simulink model "ap_12BAdapted_with_contracts_AutoPilot_SLDV"  (R2019b)
settings: Solver=FixedStepDiscrete  StartTime=0.0  StopTime=500  FixedStep=Ts  RelTol=1e-3  EnableMultiTasking=on
model workspace (MAT data in the model file):
  ContractValidatorBlocksMap : containers.Map (value not decoded)
undefined symbols (not defined in the file): beaver_b, beaver_c, beaver_mass, beaver_S, Cl0, Cl_alpha2_dpt, Cl_beta, Cl_da, Cl_da_alpha, Cl_dr, Cl_p, Cl_r, Cm0, Cm_alpha, Cm_alpha2, Cm_beta2, Cm_de, Cm_df, Cm_dpt, Cm_q, Cm_r, Cn0, Cn_beta, Cn_beta3, Cn_da, Cn_dpt3, Cn_dr, Cn_p, Cn_q, Cn_r, ContractEnsureBlock, ContractRequireBlock, Cx0, Cx_alpha, Cx_alpha2, Cx_alpha3, Cx_df, Cx_df_alpha, Cx_dpt, Cx_dpt2_alpha, Cx_dr, Cx_q, Cy0, Cy_beta, Cy_da, Cy_dr, Cy_dr_alpha, Cy_p, Cy_r, Cz0, Cz_alpha, Cz_alpha3, Cz_de, Cz_de_beta, Cz_df, Cz_df_alpha, Cz_dpt, Cz_q, d2r, fin_act_1 ... (+25)
libraries: simulink x10, sldvlib x5, cocosimLibs x3
(part 2 of 4)

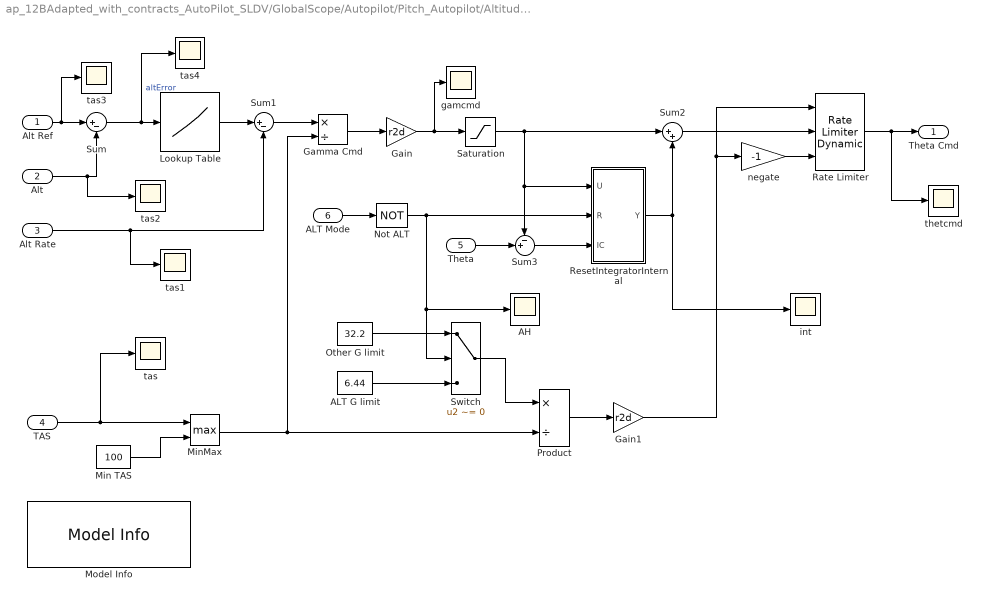
== system ap_12BAdapted_with_contracts_AutoPilot_SLDV/GlobalScope/Autopilot/Pitch_Autopilot/Altitude Mode ==
  Alt Ref : Inport  OutDataTypeStr=double  PortDimensions=1  SampleTime=1/40  Interpolate=off
  Alt : Inport  Port=2  OutDataTypeStr=double  PortDimensions=1  SampleTime=1/40  Interpolate=off
  Alt Rate : Inport  Port=3  OutDataTypeStr=double  PortDimensions=1  SampleTime=1/40  Interpolate=off
  TAS : Inport  Port=4  OutDataTypeStr=double  PortDimensions=1  SampleTime=1/40  Interpolate=off
  Theta : Inport  Port=5  OutDataTypeStr=double  PortDimensions=1  SampleTime=1/40  Interpolate=off
  ALT Mode : Inport  Port=6  OutDataTypeStr=boolean  PortDimensions=1  SampleTime=1/40  Interpolate=off
  AH : Scope
  ALT G limit : Constant  Value=6.44  OutDataTypeStr=double
  Gain : Gain  Gain=r2d
  Gain1 : Gain  Gain=r2d
  Gamma Cmd : Product  Inputs=*/  RndMeth=Zero
  Lookup Table : Lookup_n-D  NumberOfTableDimensions=1  BreakpointsForDimension1=[-544 -206 -116 -52 0 52 116 206]  Table=[-42 -26 -19 -13 0 13 19 26]  ExtrapMethod=Clip  RemoveProtectionInput=on  UseLastTableValue=on  RndMeth=Zero  FractionDataTypeStr=double  InputSameDT=on
  Min TAS : Constant  Value=100  OutDataTypeStr=double
  MinMax : MinMax  Function=max  Inputs=2  InputSameDT=on
  Model Info : simulink/Model-Wide Utilities/Model Info  Frame=on  DisplayStringWithTags=|  HorizontalTextAlignment=Left  LeftAlignmentValue=0.02
      | Altitude Mode
      | Author: %<LastModifiedBy>
      | Version: %<ModelVersion>
      | Date: %<LastModificationDate>
  Not ALT : Logic  Operator=NOT  IconShape=distinctive  AllPortsSameDT=off  OutDataTypeStr=boolean
  Other G limit : Constant  Value=32.2  OutDataTypeStr=double
  Product : Product  Inputs=*/  RndMeth=Zero
  Rate Limiter : simulink/Discontinuities/Rate Limiter Dynamic
      settings: SourceProductName=Simulink
  ResetIntegratorInternal : Subsystem
  Saturation : Saturate  UpperLimit=20  LowerLimit=-20
  Sum : Sum  Inputs=|+-
  Sum1 : Sum  Inputs=|+-
  Sum2 : Sum  Inputs=|++
  Sum3 : Sum  Inputs=-+|
  Switch : Switch  Criteria=u2 ~= 0
  gamcmd : Scope
  int : Scope
  negate : Gain  Gain=-1
  tas{,1..4} (5 alike) : Scope
  thetcmd : Scope
  Theta Cmd : Outport  OutDataTypeStr=double  PortDimensions=1  SampleTime=1/40  VectorParamsAs1DForOutWhenUnconnected=off
  wires:
  Other G limit/1 -> Switch/1
  Alt Ref/1 -> tas3/1, Sum/1
  Min TAS/1 -> MinMax/2
  Lookup Table/1 -> Sum1/1
  Rate Limiter/1 -> thetcmd/1, Theta Cmd/1
  negate/1 -> Rate Limiter/3
  MinMax/1 -> Gamma Cmd/2, Product/2
  Product/1 -> Gain1/1
  Gain1/1 -> negate/1, Rate Limiter/1
  Switch/1 -> Product/1
  ResetIntegratorInternal/1(Y) -> int/1, Sum2/2
  ALT G limit/1 -> Switch/3
  Sum2/1 -> Rate Limiter/2
  Theta/1 -> Sum3/2
  Sum/1 -> tas4/1, Lookup Table/1  "altError"
  Saturation/1 -> Sum3/1, ResetIntegratorInternal/1(U), Sum2/1
  ALT Mode/1 -> Not ALT/1
  Gain/1 -> gamcmd/1, Saturation/1
  Alt/1 -> tas2/1, Sum/2
  Sum1/1 -> Gamma Cmd/1
  Alt Rate/1 -> tas1/1, Sum1/2
  Gamma Cmd/1 -> Gain/1
  Not ALT/1 -> AH/1, Switch/2, ResetIntegratorInternal/2(R)
  Sum3/1 -> ResetIntegratorInternal/3(IC)
  TAS/1 -> tas/1, MinMax/1

== system ap_12BAdapted_with_contracts_AutoPilot_SLDV/GlobalScope/Autopilot/Pitch_Autopilot/Basic Pitch Mode ==
  note: Attitude Control using displacement, rate and integral
  Disp_Cmd : Inport  OutDataTypeStr=double  PortDimensions=1  SampleTime=1/40
  "Disp_FB " : Inport  Port=2  OutDataTypeStr=double  PortDimensions=1  SampleTime=1/40
  Rate_FB : Inport  Port=3  OutDataTypeStr=double  PortDimensions=1  SampleTime=1/40
  Engaged : Inport  Port=4  OutDataTypeStr=boolean  PortDimensions=1  SampleTime=1/40
  Cmd Limit : Saturate  UpperLimit=20  LowerLimit=-20
      settings: AttributesFormatString=%<LowerLimit> to %<UpperLimit> (deg)
  Disp Gain : Gain  Gain=2.0
  Disp Limit : Saturate  UpperLimit=20  LowerLimit=-20
      settings: AttributesFormatString=%<LowerLimit> to %<UpperLimit> (deg)
  Int Gain : Gain  Gain=0.5
  Model Info : simulink/Model-Wide Utilities/Model Info  Frame=on  DisplayStringWithTags=|  HorizontalTextAlignment=Left  LeftAlignmentValue=0.02
      | Attitude Controller
      | Author: %<LastModifiedBy>
      | Version: %<ModelVersion>
      | Date: %<LastModificationDate>
  Not engaged : Logic  Operator=NOT  IconShape=distinctive  AllPortsSameDT=off  OutDataTypeStr=boolean
  Rate Gain : Gain  Gain=2.0
  Rate Limit : Saturate  UpperLimit=3  LowerLimit=-3
      settings: AttributesFormatString=%<LowerLimit> to %<UpperLimit> (deg/sec)
  ResetIntegratorInternal : Subsystem
  Sum : Sum  Inputs=|+-
  Sum1 : Sum  Inputs=|+-
  Sum2 : Sum  Inputs=++|
  att : Scope
  q : Scope
  thet : Scope
  Surf_Cmd : Outport  OutDataTypeStr=double  PortDimensions=1  SampleTime=1/40  VectorParamsAs1DForOutWhenUnconnected=off
  wires:
  Rate Limit/1 -> Sum1/1
  ResetIntegratorInternal/1(Y) -> Sum2/1, att/1
  Sum2/1 -> Cmd Limit/1
  Disp Limit/1 -> Sum/1
  Engaged/1 -> Not engaged/1
  Cmd Limit/1 -> Surf_Cmd/1
  Disp_Cmd/1 -> Disp Limit/1
  Rate_FB/1 -> q/1, Sum1/2
  Sum1/1 -> Rate Gain/1, Int Gain/1
  Sum/1 -> Disp Gain/1
  Disp Gain/1 -> Rate Limit/1
  Rate Gain/1 -> Sum2/2
  "Disp_FB "/1 -> thet/1, Sum/2
  Not engaged/1 -> ResetIntegratorInternal/2(R)
  Int Gain/1 -> ResetIntegratorInternal/1(U)

== system ap_12BAdapted_with_contracts_AutoPilot_SLDV/GlobalScope/Autopilot/Pitch_Autopilot/Pitch Rate Feedback ==
  note: Pitch Rate Computation
  Phi : Inport
  Q : Inport  Port=2
  R : Inport  Port=3
  Gain : Gain  Gain=d2r
  Product : Product  RndMeth=Zero
  Product1 : Product  RndMeth=Zero
  Sum3 : Sum  Inputs=|++
  cos : Trigonometry  Operator=cos  OutputSignalType=real
  q : Scope
  sin : Trigonometry  OutputSignalType=real
  Pitch Rate : Outport  VectorParamsAs1DForOutWhenUnconnected=off
  wires:
  Phi/1 -> Gain/1
  Product/1 -> Sum3/2
  sin/1 -> Product/1
  R/1 -> Product/2
  Gain/1 -> sin/1, cos/1
  Product1/1 -> Sum3/1
  cos/1 -> Product1/1
  Q/1 -> Product1/2
  Sum3/1 -> q/1, Pitch Rate/1

== system ap_12BAdapted_with_contracts_AutoPilot_SLDV/GlobalScope/Autopilot/Pitch_Autopilot/Pitch Reference ==
  note: Pitch Reference
  Theta : Inport
  AP Eng : Inport  Port=2
  Pitch Wheel : Inport  Port=3
  Not engaged : Logic  Operator=NOT  IconShape=distinctive  AllPortsSameDT=off  OutDataTypeStr=boolean
  Sum3 : Sum  Inputs=|++
  latch : Subsystem
  Theta Ref : Outport  VectorParamsAs1DForOutWhenUnconnected=off
  wires:
  Not engaged/1 -> latch/2(E)
  latch/1(y) -> Sum3/1
  Theta/1 -> latch/1(u)
  AP Eng/1 -> Not engaged/1
  Sum3/1 -> Theta Ref/1
  Pitch Wheel/1 -> Sum3/2

== system ap_12BAdapted_with_contracts_AutoPilot_SLDV/GlobalScope/Autopilot/Roll_Autopilot/Basic Roll Mode ==
  note: Attitude Control using displacement, rate and integral
  Disp_Cmd : Inport  OutDataTypeStr=double  PortDimensions=1
  "Disp_FB " : Inport  Port=2  OutDataTypeStr=double  PortDimensions=1  SampleTime=1/40
  Rate_FB : Inport  Port=3  OutDataTypeStr=double  PortDimensions=1  SampleTime=1/40
  Engaged : Inport  Port=4  OutDataTypeStr=boolean  PortDimensions=1  SampleTime=1/40
  Cmd Limit : Saturate  UpperLimit=15  LowerLimit=-15
      settings: AttributesFormatString=%<LowerLimit> to %<UpperLimit> (deg)
  Disp Gain : Gain  Gain=1.0
  Disp Limit : Saturate  UpperLimit=30  LowerLimit=-30
      settings: AttributesFormatString=%<LowerLimit> to %<UpperLimit> (deg)
  Int Gain : Gain  Gain=1.0
  Model Info : simulink/Model-Wide Utilities/Model Info  Frame=on  DisplayStringWithTags=|  HorizontalTextAlignment=Left  LeftAlignmentValue=0.02
      | Attitude Controller
      | Author: %<LastModifiedBy>
      | Version: %<ModelVersion>
      | Date: %<LastModificationDate>
  Not engaged : Logic  Operator=NOT  IconShape=distinctive  AllPortsSameDT=off  OutDataTypeStr=boolean
  Rate Gain : Gain  Gain=3.0
  Rate Limit : Saturate  UpperLimit=6  LowerLimit=-6
      settings: AttributesFormatString=%<LowerLimit> to %<UpperLimit> (deg/sec)
  ResetIntegratorInternal : Subsystem
  Scope : Scope
  Scope1 : Scope
  Scope2 : Scope
  Sum : Sum  Inputs=|+-
  Sum1 : Sum  Inputs=|+-
  Sum2 : Sum  Inputs=++|
  Surf_Cmd : Outport  OutDataTypeStr=double  PortDimensions=1  SampleTime=1/40  VectorParamsAs1DForOutWhenUnconnected=off
  wires:
  Engaged/1 -> Not engaged/1
  Disp_Cmd/1 -> Disp Limit/1
  Rate Limit/1 -> Sum1/1
  ResetIntegratorInternal/1(Y) -> Sum2/1, Scope/1
  Not engaged/1 -> ResetIntegratorInternal/2(R)
  Rate_FB/1 -> Sum1/2
  Sum1/1 -> Int Gain/1, Scope1/1, Rate Gain/1
  Cmd Limit/1 -> Scope2/1, Surf_Cmd/1
  Rate Gain/1 -> Sum2/2
  Disp Gain/1 -> Rate Limit/1
  Sum/1 -> Disp Gain/1
  "Disp_FB "/1 -> Sum/2
  Disp Limit/1 -> Sum/1
  Sum2/1 -> Cmd Limit/1
  Int Gain/1 -> ResetIntegratorInternal/1(U)

== system ap_12BAdapted_with_contracts_AutoPilot_SLDV/GlobalScope/Autopilot/Roll_Autopilot/Heading Mode ==
  Psi Ref : Inport  OutDataTypeStr=double  PortDimensions=1  SampleTime=1/40  Interpolate=off
  Psi : Inport  Port=2  OutDataTypeStr=double  PortDimensions=1  SampleTime=1/40  Interpolate=off
  TAS : Inport  Port=3  OutDataTypeStr=double  PortDimensions=1  SampleTime=1/40  Interpolate=off
  Disp Gain : Gain  Gain=0.015
  Model Info : simulink/Model-Wide Utilities/Model Info  Frame=on  DisplayStringWithTags=|  HorizontalTextAlignment=Left  LeftAlignmentValue=0.02
      | Heading Mode
      | Author: %<LastModifiedBy>
      | Version: %<ModelVersion>
      | Date: %<LastModificationDate>
  Product : Product  RndMeth=Zero
  angle diff : Subsystem
  Phi Cmd : Outport  OutDataTypeStr=double  PortDimensions=1  SampleTime=1/40  VectorParamsAs1DForOutWhenUnconnected=off
  wires:
  Psi Ref/1 -> angle diff/1(plus)
  angle diff/1(diff) -> Disp Gain/1  "hdgError"
  TAS/1 -> Product/2
  Disp Gain/1 -> Product/1
  Psi/1 -> angle diff/2(minus)
  Product/1 -> Phi Cmd/1

== system ap_12BAdapted_with_contracts_AutoPilot_SLDV/GlobalScope/Autopilot/Roll_Autopilot/Roll Reference ==
  note: Roll Reference
  Phi : Inport
  AP eng : Inport  Port=2
  Turn Knob : Inport  Port=3
  Abs : Abs
  Not engaged : Logic  Operator=NOT  IconShape=distinctive  AllPortsSameDT=off  OutDataTypeStr=boolean
  Ref Threshold : RelationalOperator  OutDataTypeStr=boolean  RndMeth=Nearest  InputSameDT=on
  Ref Threshold1 : RelationalOperator  Operator=<=  OutDataTypeStr=boolean  RndMeth=Nearest  InputSameDT=on
  TK Threshold : RelationalOperator  Operator=<  OutDataTypeStr=boolean  RndMeth=Nearest  InputSameDT=on
  TK switch : Switch  Criteria=u2 ~= 0
  latch : Subsystem
  minus six : Constant  Value=-6
  or : Logic  Operator=OR  IconShape=distinctive  OutDataTypeStr=boolean
  ref switch : Switch  Criteria=u2 ~= 0
  six : Constant  Value=6
  three : Constant  Value=3  OutDataTypeStr=double
  zero : Constant  Value=0
  Phi Ref : Outport  VectorParamsAs1DForOutWhenUnconnected=off
  wires:
  minus six/1 -> Ref Threshold1/2
  Ref Threshold1/1 -> or/2
  Ref Threshold/1 -> or/1
  or/1 -> ref switch/2
  zero/1 -> ref switch/3
  six/1 -> Ref Threshold/2
  TK switch/1 -> Phi Ref/1
  AP eng/1 -> Not engaged/1
  Phi/1 -> Ref Threshold1/1, Ref Threshold/1, ref switch/1
  Abs/1 -> TK Threshold/1
  three/1 -> TK Threshold/2
  Turn Knob/1 -> Abs/1, TK switch/3
  TK Threshold/1 -> TK switch/2
  latch/1(y) -> TK switch/1
  ref switch/1 -> latch/1(u)
  Not engaged/1 -> latch/2(E)

== system ap_12BAdapted_with_contracts_AutoPilot_SLDV/GlobalScope/Autopilot/Yaw_damper/Basic Yaw Damper ==
  note: Basic Yaw Damper
  "Phi " : Inport
  R : Inport  Port=2
  TAS : Inport  Port=3
  Constant : Constant  Value=100
  MinMax : MinMax  Function=max  Inputs=2
  Model Info : simulink/Model-Wide Utilities/Model Info  Frame=on  DisplayStringWithTags=|  HorizontalTextAlignment=Left  LeftAlignmentValue=0.02
      | Yaw Damper
      | Author: %<LastModifiedBy>
      | Date: %<LastModificationDate>
      | Model Version: %<ModelVersion>
  Product : Product  Inputs=*/  RndMeth=Zero
  Rate Gain : Gain  Gain=1.0
  Rud Limit : Saturate  UpperLimit=25  LowerLimit=-25
      settings: AttributesFormatString=%<LowerLimit> to %<UpperLimit> (deg)
  Sum1 : Sum  Inputs=|+-
  gravity : Gain  Gain=32.2
  sin : Trigonometry
  Rud Cmd : Outport  VectorParamsAs1DForOutWhenUnconnected=off
  wires:
  R/1 -> Sum1/2
  Sum1/1 -> Rate Gain/1  "yawRate"
  Rud Limit/1 -> Rud Cmd/1
  Rate Gain/1 -> Rud Limit/1
  "Phi "/1 -> sin/1
  sin/1 -> gravity/1
  Product/1 -> Sum1/1
  gravity/1 -> Product/1
  MinMax/1 -> Product/2
  TAS/1 -> MinMax/1
  Constant/1 -> MinMax/2

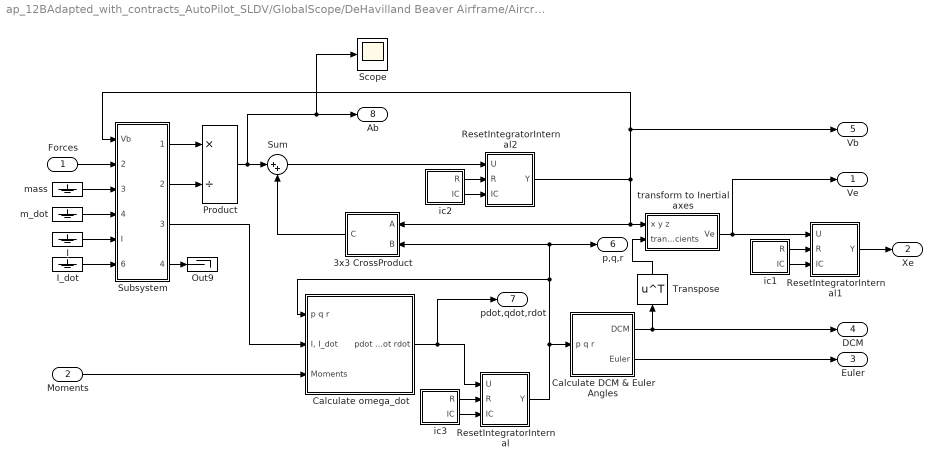
== system ap_12BAdapted_with_contracts_AutoPilot_SLDV/GlobalScope/DeHavilland Beaver Airframe/Aircraft Dynamics/6DoF (Quaternion) ==
  Forces : Inport
  Moments : Inport  Port=2
  3x3 CrossProduct : Subsystem
  Calculate DCM & Euler Angles : Subsystem
  Calculate omega_dot : Subsystem
  I : Ground
  I_dot : Ground
  Out9 : Terminator
  Product : Product  Inputs=*/  SaturateOnIntegerOverflow=on  OutDataTypeStr=Inherit: Same as first input
  ResetIntegratorInternal : Subsystem
  ResetIntegratorInternal1 : Subsystem
  ResetIntegratorInternal2 : Subsystem
  Scope : Scope
  Subsystem : Subsystem
  Sum : Sum  Inputs=|++  SaturateOnIntegerOverflow=on
  Transpose : Math  Operator=transpose  SaturateOnIntegerOverflow=on
  ic1 : Subsystem
  ic2 : Subsystem
  ic3 : Subsystem
  m_dot : Ground
  mass : Ground
  "transform to Inertial axes " : Subsystem
  Ve : Outport  VectorParamsAs1DForOutWhenUnconnected=off
  Xe : Outport  Port=2  VectorParamsAs1DForOutWhenUnconnected=off
  Euler : Outport  Port=3  VectorParamsAs1DForOutWhenUnconnected=off
  DCM : Outport  Port=4  VectorParamsAs1DForOutWhenUnconnected=off
  Vb : Outport  Port=5  VectorParamsAs1DForOutWhenUnconnected=off
  p,q,r : Outport  Port=6  VectorParamsAs1DForOutWhenUnconnected=off
  pdot,qdot,rdot : Outport  Port=7  VectorParamsAs1DForOutWhenUnconnected=off
  Ab : Outport  Port=8  VectorParamsAs1DForOutWhenUnconnected=off
  wires:
  Subsystem/1("forces ") -> Product/1
  I_dot/1 -> Subsystem/6(I_dot)
  I/1 -> Subsystem/5(I)
  Calculate omega_dot/1(pdot qdot rdot) -> pdot,qdot,rdot/1, ResetIntegratorInternal/1(U)
  Subsystem/4(Out9) -> Out9/1
  m_dot/1 -> Subsystem/4(m_dot)
  Subsystem/2(mass) -> Product/2
  mass/1 -> Subsystem/3("mass ")
  Transpose/1 -> "transform to Inertial axes "/2(transform coefficients)
  Calculate DCM & Euler Angles/1(DCM) -> DCM/1, Transpose/1
  Product/1 -> Scope/1, Ab/1, Sum/1
  Forces/1 -> Subsystem/2(forces)
  Moments/1 -> Calculate omega_dot/3(Moments)
  ResetIntegratorInternal1/1(Y) -> Xe/1
  Sum/1 -> ResetIntegratorInternal2/1(U)
  3x3 CrossProduct/1(C) -> Sum/2
  Calculate DCM & Euler Angles/2(Euler) -> Euler/1
  Subsystem/3("inertia, 0") -> Calculate omega_dot/2("I, I_dot")
  "transform to Inertial axes "/1(Ve) -> ResetIntegratorInternal1/1(U), Ve/1
  ResetIntegratorInternal/1(Y) -> Calculate DCM & Euler Angles/1(p q r), 3x3 CrossProduct/2(B), p,q,r/1, Calculate omega_dot/1(p q r)
  ic3/1(R) -> ResetIntegratorInternal/2(R)
  ic3/2(IC) -> ResetIntegratorInternal/3(IC)
  ic1/1(R) -> ResetIntegratorInternal1/2(R)
  ic1/2(IC) -> ResetIntegratorInternal1/3(IC)
  ic2/1(R) -> ResetIntegratorInternal2/2(R)
  ic2/2(IC) -> ResetIntegratorInternal2/3(IC)
  ResetIntegratorInternal2/1(Y) -> Subsystem/1(Vb), Vb/1, 3x3 CrossProduct/1(A), "transform to Inertial axes "/1(x y z)

== system ap_12BAdapted_with_contracts_AutoPilot_SLDV/GlobalScope/DeHavilland Beaver Airframe/Aircraft Dynamics/Total Forces and Moments ==
  EnvirBus : Inport
  Pilot : Inport  Port=2
  DCM : Inport  Port=3
  FltParams : Inport  Port=4
  Actuators : Subsystem
  Aerodynamics : Subsystem
  Bus Selector4 : BusSelector  OutputSignals=rho,g
  "Engine " : Subsystem
  Forces and Moments : Subsystem
  "Gravity " : Subsystem
  "Pilot " : InportShadow  Port=2
  Sum : Sum  Inputs=|++  SaturateOnIntegerOverflow=on  InputSameDT=on  OutDataTypeStr=Inherit: Same as first input
  Total Force : Outport  VectorParamsAs1DForOutWhenUnconnected=off
  Total Moment : Outport  Port=2  VectorParamsAs1DForOutWhenUnconnected=off
  wires:
  Forces and Moments/1(XYZ) -> Sum/1
  "Engine "/1(Engine Coefficients) -> Forces and Moments/3(Engine Coefficients)
  "Gravity "/1(Fgrav) -> Sum/2
  Aerodynamics/1(Aero Coefficients) -> Forces and Moments/1(Aero Coefficients)
  Pilot/1 -> Actuators/1(Pilot)
  Bus Selector4/1 -> "Engine "/3(rho)  "<rho>"
  DCM/1 -> "Gravity "/2(DCM)
  Bus Selector4/2 -> "Gravity "/1(g)  "<g>"
  Sum/1 -> Total Force/1  "Ftot"
  Forces and Moments/2(LMN) -> Total Moment/1  "Mtot"
  "Pilot "/1 -> "Engine "/2(Pilot)
  FltParams/1 -> Forces and Moments/2(Fltparams), "Engine "/1(Fltparams), Aerodynamics/2(FltParams)
  Actuators/1(uaero-out) -> Aerodynamics/1(Uaero)
  EnvirBus/1 -> Bus Selector4/1

== system ap_12BAdapted_with_contracts_AutoPilot_SLDV/GlobalScope/DeHavilland Beaver Airframe/Calculate Parameters/ Incidence, Sideslip, & Airspeed ==
  Vb : Inport
  Airspeed : Sqrt  AlgorithmType=Newton-Raphson  SaturateOnIntegerOverflow=on
  Incidence : Trigonometry  Operator=atan2
  Product : Product  Inputs=*/  SaturateOnIntegerOverflow=on  OutDataTypeStr=Inherit: Same as first input
  Sideslip : Trigonometry  Operator=asin
  Subsystem : Subsystem
  Subsystem1 : Subsystem
  dot : Subsystem
  Alpha : Outport  VectorParamsAs1DForOutWhenUnconnected=off
  Beta : Outport  Port=2  VectorParamsAs1DForOutWhenUnconnected=off
  V : Outport  Port=3  VectorParamsAs1DForOutWhenUnconnected=off
  wires:
  Sideslip/1 -> Beta/1
  Subsystem1/1(v) -> Product/1
  Product/1 -> Sideslip/1
  Subsystem/1(w) -> Incidence/1
  Subsystem/2(U) -> Incidence/2
  dot/1(dot) -> Airspeed/1
  Airspeed/1 -> V/1, Product/2
  Incidence/1 -> Alpha/1
  Vb/1 -> Subsystem/1(V), dot/1(Vb), Subsystem1/1(V)

== system ap_12BAdapted_with_contracts_AutoPilot_SLDV/GlobalScope/DeHavilland Beaver Airframe/Calculate Parameters/Dynamic Pressure ==
  Velocity : Inport
  Air Density : Inport  Port=2
  1/2rhoV^2 : Gain  Gain=0.5  SaturateOnIntegerOverflow=on  OutDataTypeStr=Inherit: Same as input  ParamDataTypeStr=Inherit: Same as input
  Product2 : Product  SaturateOnIntegerOverflow=on  InputSameDT=on  OutDataTypeStr=Inherit: Same as first input
  dot : Subsystem
  qbar : Outport  VectorParamsAs1DForOutWhenUnconnected=off
  wires:
  1/2rhoV^2/1 -> qbar/1
  Air Density/1 -> Product2/2
  dot/1(dot) -> Product2/1
  Product2/1 -> 1/2rhoV^2/1
  Velocity/1 -> dot/1(V)

== system ap_12BAdapted_with_contracts_AutoPilot_SLDV/GlobalScope/Sensors/Air Data Sensor/ Incidence, Sideslip, & Airspeed ==
  Vb : Inport
  Airspeed : Sqrt  AlgorithmType=Newton-Raphson  SaturateOnIntegerOverflow=on
  Gain : Gain  Gain=180/pi
  Gain1 : Gain  Gain=180/pi
  Incidence : Trigonometry  Operator=atan2
  Product : Product  Inputs=*/  SaturateOnIntegerOverflow=on  OutDataTypeStr=Inherit: Same as first input
  Scope : Scope
  Scope1 : Scope
  Sideslip : Trigonometry  Operator=asin
  Subsystem : Subsystem
  Subsystem1 : Subsystem
  dot : Subsystem
  Alpha : Outport  VectorParamsAs1DForOutWhenUnconnected=off
  Beta : Outport  Port=2  VectorParamsAs1DForOutWhenUnconnected=off
  V : Outport  Port=3  VectorParamsAs1DForOutWhenUnconnected=off
  wires:
  Sideslip/1 -> Gain1/1, Beta/1
  Subsystem1/1(v) -> Product/1
  Product/1 -> Sideslip/1
  Subsystem/1(w) -> Incidence/1
  Subsystem/2(U) -> Incidence/2
  dot/1(dot) -> Airspeed/1
  Airspeed/1 -> V/1, Product/2
  Incidence/1 -> Gain/1, Alpha/1
  Vb/1 -> Subsystem/1(V), dot/1(Vb), Subsystem1/1(V)
  Gain/1 -> Scope/1
  Gain1/1 -> Scope1/1

== system ap_12BAdapted_with_contracts_AutoPilot_SLDV/GlobalScope/Sensors/Air Data Sensor/ic1 ==
  u : Inport
  ic : Inport  Port=2
  Constant : Constant
  Switch : Switch  Criteria=u2 ~= 0
  Unit Delay : UnitDelay  SampleTime=-1  HasFrameUpgradeWarning=on
  y : Outport  VectorParamsAs1DForOutWhenUnconnected=off
  wires:
  Switch/1 -> y/1
  u/1 -> Switch/1
  ic/1 -> Switch/3
  Constant/1 -> Unit Delay/1
  Unit Delay/1 -> Switch/2

== system ap_12BAdapted_with_contracts_AutoPilot_SLDV/GlobalScope/Sensors/Air Data Sensor/ic2 ==
  u : Inport
  ic : Inport  Port=2
  Constant : Constant
  Switch : Switch  Criteria=u2 ~= 0
  Unit Delay : UnitDelay  SampleTime=-1  HasFrameUpgradeWarning=on
  y : Outport  VectorParamsAs1DForOutWhenUnconnected=off
  wires:
  ic/1 -> Switch/3
  u/1 -> Switch/1
  Switch/1 -> y/1
  Constant/1 -> Unit Delay/1
  Unit Delay/1 -> Switch/2

== system ap_12BAdapted_with_contracts_AutoPilot_SLDV/GlobalScope/Sensors/Air Data Sensor/ic3 ==
  u : Inport
  ic : Inport  Port=2
  Constant1 : Constant
  Switch : Switch  Criteria=u2 ~= 0
  Unit Delay1 : UnitDelay  SampleTime=-1  HasFrameUpgradeWarning=on
  y : Outport  VectorParamsAs1DForOutWhenUnconnected=off
  wires:
  ic/1 -> Switch/3
  u/1 -> Switch/1
  Switch/1 -> y/1
  Constant1/1 -> Unit Delay1/1
  Unit Delay1/1 -> Switch/2

== system ap_12BAdapted_with_contracts_AutoPilot_SLDV/GlobalScope/Sensors/Inertial Data Sensor/ic ==
  u : Inport
  ic : Inport  Port=2
  Constant : Constant
  Switch : Switch  Criteria=u2 ~= 0
  Unit Delay : UnitDelay  SampleTime=-1  HasFrameUpgradeWarning=on
  y : Outport  VectorParamsAs1DForOutWhenUnconnected=off
  wires:
  Switch/1 -> y/1
  u/1 -> Switch/1
  ic/1 -> Switch/3
  Constant/1 -> Unit Delay/1
  Unit Delay/1 -> Switch/2

== system ap_12BAdapted_with_contracts_AutoPilot_SLDV/GlobalScope/Sensors/Inertial Data Sensor/ic1 ==
  u : Inport
  ic : Inport  Port=2
  Constant : Constant
  Switch : Switch  Criteria=u2 ~= 0
  Unit Delay : UnitDelay  SampleTime=-1  HasFrameUpgradeWarning=on
  y : Outport  VectorParamsAs1DForOutWhenUnconnected=off
  wires:
  ic/1 -> Switch/3
  u/1 -> Switch/1
  Switch/1 -> y/1
  Constant/1 -> Unit Delay/1
  Unit Delay/1 -> Switch/2

== system ap_12BAdapted_with_contracts_AutoPilot_SLDV/GlobalScope/Sensors/Inertial Data Sensor/ic2 ==
  u : Inport
  ic : Inport  Port=2
  Constant : Constant
  Switch : Switch  Criteria=u2 ~= 0
  Unit Delay : UnitDelay  SampleTime=-1  HasFrameUpgradeWarning=on
  y : Outport  VectorParamsAs1DForOutWhenUnconnected=off
  wires:
  Switch/1 -> y/1
  u/1 -> Switch/1
  ic/1 -> Switch/3
  Constant/1 -> Unit Delay/1
  Unit Delay/1 -> Switch/2

== system ap_12BAdapted_with_contracts_AutoPilot_SLDV/GlobalScope/Sensors/Inertial Data Sensor/ic3 ==
  u : Inport
  ic : Inport  Port=2
  Constant : Constant
  Switch : Switch  Criteria=u2 ~= 0
  Unit Delay : UnitDelay  SampleTime=-1  HasFrameUpgradeWarning=on
  y : Outport  VectorParamsAs1DForOutWhenUnconnected=off
  wires:
  ic/1 -> Switch/3
  u/1 -> Switch/1
  Switch/1 -> y/1
  Constant/1 -> Unit Delay/1
  Unit Delay/1 -> Switch/2

== system ap_12BAdapted_with_contracts_AutoPilot_SLDV/GlobalScope/Autopilot/Pitch_Autopilot/Altitude Mode/ResetIntegratorInternal ==
  note: ic
  note: Level Reset Integration With Saturation
      | y(n) = y(n-1) + K*Ts*u(n-1)
  U : Inport
  R : Inport  Port=2
  IC : Inport  Port=3
  Constant : Constant  Value=0.2
  Constant1 : Constant  Value=Ts
  Product : Product  RndMeth=Zero
  Product1 : Product  RndMeth=Zero
  Saturation : Saturate  UpperLimit=20  LowerLimit=-20
  Sum3 : Sum
  Switch : Switch  Criteria=u2 ~= 0
  Switch1 : Switch  Criteria=u2 ~= 0
  X : UnitDelay  SampleTime=Ts  HasFrameUpgradeWarning=on
  Y : Outport  VectorParamsAs1DForOutWhenUnconnected=off
  wires:
  Product1/1 -> Sum3/1
  U/1 -> Product1/2
  Sum3/1 -> Switch1/3
  Product/1 -> Product1/1
  Switch/1 -> Saturation/1
  IC/1 -> Switch1/1, Switch/1
  Constant1/1 -> Product/2  "deltaT"
  Switch1/1 -> X/1
  Constant/1 -> Product/1  "gain"
  Saturation/1 -> Y/1, Sum3/2
  R/1 -> Switch1/2, Switch/2
  X/1 -> Switch/3

== system ap_12BAdapted_with_contracts_AutoPilot_SLDV/GlobalScope/Autopilot/Pitch_Autopilot/Basic Pitch Mode/ResetIntegratorInternal ==
  note: ic
  note: Level Reset Integration With Saturation
      | y(n) = y(n-1) + K*Ts*u(n-1)
  U : Inport
  R : Inport  Port=2
  Constant : Constant  Value=1.0
  Constant1 : Constant  Value=Ts
  Constant2 : Constant  Value=0.0
  Product : Product  RndMeth=Zero
  Product1 : Product  RndMeth=Zero
  Saturation : Saturate  UpperLimit=5  LowerLimit=-5
  Sum3 : Sum
  Switch : Switch  Criteria=u2 ~= 0
  Switch1 : Switch  Criteria=u2 ~= 0
  X : UnitDelay  SampleTime=Ts  HasFrameUpgradeWarning=on
  Y : Outport  VectorParamsAs1DForOutWhenUnconnected=off
  wires:
  Product1/1 -> Sum3/1
  U/1 -> Product1/2
  Sum3/1 -> Switch1/3
  Product/1 -> Product1/1
  Switch/1 -> Saturation/1
  Constant2/1 -> Switch1/1, Switch/1
  Constant1/1 -> Product/2  "deltaT"
  Switch1/1 -> X/1
  Constant/1 -> Product/1  "gain"
  Saturation/1 -> Y/1, Sum3/2
  R/1 -> Switch1/2, Switch/2
  X/1 -> Switch/3

== system ap_12BAdapted_with_contracts_AutoPilot_SLDV/GlobalScope/Autopilot/Pitch_Autopilot/Pitch Reference/latch ==
  note: Xold
  note: Enable
  u : Inport
  E : Inport  Port=2
  Enable : Switch  Criteria=u2 ~= 0  OutDataTypeStr=Inherit: Inherit via back propagation  ZeroCross=off
  FixPt Unit Delay1 : UnitDelay  SampleTime=Ts
  y : Outport  VectorParamsAs1DForOutWhenUnconnected=off
  wires:
  FixPt Unit Delay1/1 -> y/1, Enable/3
  Enable/1 -> FixPt Unit Delay1/1  "Xnew"
  E/1 -> Enable/2
  u/1 -> Enable/1

== system ap_12BAdapted_with_contracts_AutoPilot_SLDV/GlobalScope/Autopilot/Roll_Autopilot/Basic Roll Mode/ResetIntegratorInternal ==
  note: ic
  note: Level Reset Integration With Saturation
      | y(n) = y(n-1) + K*Ts*u(n-1)
  U : Inport
  R : Inport  Port=2
  Constant : Constant  Value=1.0
  Constant1 : Constant  Value=Ts
  Constant2 : Constant  Value=0.0
  Product : Product  RndMeth=Zero
  Product1 : Product  RndMeth=Zero
  Saturation : Saturate  UpperLimit=5  LowerLimit=-5
  Sum3 : Sum
  Switch : Switch  Criteria=u2 ~= 0
  Switch1 : Switch  Criteria=u2 ~= 0
  X : UnitDelay  SampleTime=Ts  HasFrameUpgradeWarning=on
  Y : Outport  VectorParamsAs1DForOutWhenUnconnected=off
  wires:
  Product1/1 -> Sum3/1
  U/1 -> Product1/2
  Sum3/1 -> Switch1/3
  Product/1 -> Product1/1
  Switch/1 -> Saturation/1
  Constant2/1 -> Switch1/1, Switch/1
  Constant1/1 -> Product/2  "deltaT"
  Switch1/1 -> X/1
  Constant/1 -> Product/1  "gain"
  Saturation/1 -> Y/1, Sum3/2
  R/1 -> Switch1/2, Switch/2
  X/1 -> Switch/3

== system ap_12BAdapted_with_contracts_AutoPilot_SLDV/GlobalScope/Autopilot/Roll_Autopilot/Heading Mode/angle diff ==
  plus : Inport  OutDataTypeStr=double
  minus : Inport  Port=2  OutDataTypeStr=double
  abs : Abs  ZeroCross=off
  constant : Constant  Value=180
  constant1 : Constant  Value=360
  floor : Rounding
  product : Product  RndMeth=Zero  InputSameDT=on  OutDataTypeStr=Inherit: Same as first input
  product1 : Product  Inputs=*/  RndMeth=Zero  InputSameDT=on  OutDataTypeStr=Inherit: Same as first input
  product2 : Product  RndMeth=Zero  InputSameDT=on  OutDataTypeStr=Inherit: Same as first input
  signum : Signum  ZeroCross=off
  sum : Sum  Inputs=|+-  RndMeth=Zero  InputSameDT=on  OutDataTypeStr=Inherit: Same as first input
  sum1 : Sum  Inputs=|+-  RndMeth=Zero  InputSameDT=on  OutDataTypeStr=Inherit: Same as first input
  sum2 : Sum  Inputs=|++  RndMeth=Zero  InputSameDT=on  OutDataTypeStr=Inherit: Same as first input
  diff : Outport  VectorParamsAs1DForOutWhenUnconnected=off
  wires:
  product2/1 -> product/2
  product/1 -> sum1/2
  sum2/1 -> product1/1
  constant/1 -> sum2/2
  sum1/1 -> diff/1
  signum/1 -> product/1
  floor/1 -> product2/1
  minus/1 -> sum/2
  plus/1 -> sum/1
  product1/1 -> floor/1
  sum/1 -> sum1/1, abs/1, signum/1
  abs/1 -> sum2/1
  constant1/1 -> product2/2, product1/2

== system ap_12BAdapted_with_contracts_AutoPilot_SLDV/GlobalScope/Autopilot/Roll_Autopilot/Roll Reference/latch ==
  note: Xold
  note: Enable
  u : Inport
  E : Inport  Port=2
  Enable : Switch  Criteria=u2 ~= 0  OutDataTypeStr=Inherit: Inherit via back propagation  ZeroCross=off
  FixPt Unit Delay1 : UnitDelay  SampleTime=Ts
  y : Outport  VectorParamsAs1DForOutWhenUnconnected=off
  wires:
  FixPt Unit Delay1/1 -> y/1, Enable/3
  Enable/1 -> FixPt Unit Delay1/1  "Xnew"
  E/1 -> Enable/2
  u/1 -> Enable/1

== system ap_12BAdapted_with_contracts_AutoPilot_SLDV/GlobalScope/DeHavilland Beaver Airframe/Aircraft Dynamics/6DoF (Quaternion)/3x3 CrossProduct ==
  A : Inport
  B : Inport  Port=2
  "A " : InportShadow
  "B " : InportShadow  Port=2
  Subsystem : Subsystem
  Subsystem1 : Subsystem
  Sum : Sum  Inputs=+|-  SaturateOnIntegerOverflow=on  InputSameDT=on  OutDataTypeStr=Inherit: Same as first input
  C : Outport  VectorParamsAs1DForOutWhenUnconnected=off
  wires:
  "A "/1 -> Subsystem1/1(A)
  Subsystem/1(Out1) -> Sum/1
  B/1 -> Subsystem/2(B)
  Sum/1 -> C/1
  "B "/1 -> Subsystem1/2(B)
  Subsystem1/1(Out1) -> Sum/2
  A/1 -> Subsystem/1(A)

== system ap_12BAdapted_with_contracts_AutoPilot_SLDV/GlobalScope/DeHavilland Beaver Airframe/Aircraft Dynamics/6DoF (Quaternion)/Calculate DCM & Euler Angles ==
  p q r : Inport
  Initial Euler Angles : Constant  Value="[0    0.1303    1.9722]"
  Quaternions to Direction Cosine Matrix : Subsystem
  Quaternions to Rotation Angles (ZYX) : Subsystem
  ResetIntegratorInternal1 : Subsystem
  Rotation Angles to Quats (ZYX) : Subsystem
  Selector : Selector  InputPortWidth=3  IndexOptions=Index vector (dialog)  Indices=[3 2 1]  OutputSizes=1
  Selector1 : Selector  InputPortWidth=3  IndexOptions=Index vector (dialog)  Indices=[3 2 1]  OutputSizes=1
  ic3 : Subsystem
  qd : Subsystem
  DCM : Outport  VectorParamsAs1DForOutWhenUnconnected=off
  Euler : Outport  Port=2  VectorParamsAs1DForOutWhenUnconnected=off
  wires:
  Selector1/1 -> Rotation Angles to Quats (ZYX)/1("R1, R2, R3")
  Selector/1 -> Euler/1
  Quaternions to Rotation Angles (ZYX)/1(R1,R2,R3) -> Selector/1
  Quaternions to Direction Cosine Matrix/1(DCM) -> DCM/1
  p q r/1 -> qd/1(p q r)
  Initial Euler Angles/1 -> Selector1/1
  ResetIntegratorInternal1/1(Y) -> Quaternions to Direction Cosine Matrix/1(Quat), qd/2(q0 q1 q2 q3), Quaternions to Rotation Angles (ZYX)/1(q)
  qd/1(qdot) -> ResetIntegratorInternal1/1(U)
  ic3/1(R) -> ResetIntegratorInternal1/2(R)
  ic3/2(IC) -> ResetIntegratorInternal1/3(IC)
  Rotation Angles to Quats (ZYX)/1(Quat) -> ic3/1(ic)

== system ap_12BAdapted_with_contracts_AutoPilot_SLDV/GlobalScope/DeHavilland Beaver Airframe/Aircraft Dynamics/6DoF (Quaternion)/Calculate omega_dot ==
  p q r : Inport
  "I, I_dot" : Inport  Port=2
  Moments : Inport  Port=3
  3x3 CrossProduct : Subsystem
  I x w : Subsystem
  I x w1 : Subsystem
  Product2 : Product  Inputs=*/  Multiplication=Matrix(*)  SaturateOnIntegerOverflow=on  OutDataTypeStr=Inherit: Same as first input
  Reshape : Reshape
  Reshape1 : Reshape  OutputDimensionality=Row vector (2-D)
  Selector : Selector  NumberOfDimensions=2  InputPortWidth=2  IndexOptions=Index vector (dialog),Select all  Indices=1:3,-1  OutputSizes=1
  Selector1 : Selector  NumberOfDimensions=2  InputPortWidth=2  IndexOptions=Index vector (dialog),Select all  Indices=4:6,-1  OutputSizes=1
  Selector2 : Selector  NumberOfDimensions=2  InputPortWidth=2  IndexOptions=Index vector (dialog),Select all  Indices=1:3,-1  OutputSizes=1
  Sum2 : Sum  Inputs=+--  SaturateOnIntegerOverflow=on
  pdot qdot rdot : Outport  VectorParamsAs1DForOutWhenUnconnected=off
  wires:
  Reshape1/1 -> Product2/1
  I x w/1(I * w) -> 3x3 CrossProduct/2(B)
  3x3 CrossProduct/1(C) -> Sum2/3
  Selector1/1 -> I x w1/1(I_dot)
  I x w1/1(Id * w) -> Sum2/2
  Moments/1 -> Sum2/1
  Sum2/1 -> Reshape1/1
  Product2/1 -> Reshape/1
  p q r/1 -> I x w/1(p q r), I x w1/2(p q r), 3x3 CrossProduct/1(A)
  "I, I_dot"/1 -> Selector2/1, Selector/1, Selector1/1
  Selector2/1 -> Product2/2
  Selector/1 -> I x w/2(Inertia)
  Reshape/1 -> pdot qdot rdot/1

== system ap_12BAdapted_with_contracts_AutoPilot_SLDV/GlobalScope/DeHavilland Beaver Airframe/Aircraft Dynamics/6DoF (Quaternion)/ResetIntegratorInternal ==
  note: ic
  note: Level Reset Integration With Saturation
      | y(n) = y(n-1) + K*Ts*u(n-1)
  U : Inport
  R : Inport  Port=2
  IC : Inport  Port=3
  Constant : Constant  Value=1.0
  Constant1 : Constant  Value=Ts
  Product : Product  RndMeth=Zero
  Product1 : Product  RndMeth=Zero
  Sum3 : Sum
  Switch : Switch  Criteria=u2 ~= 0
  Switch1 : Switch  Criteria=u2 ~= 0
  X : UnitDelay  SampleTime=Ts  HasFrameUpgradeWarning=on
  Y : Outport  VectorParamsAs1DForOutWhenUnconnected=off
  wires:
  Product1/1 -> Sum3/1
  U/1 -> Product1/2
  Sum3/1 -> Switch1/3
  Product/1 -> Product1/1
  IC/1 -> Switch1/1, Switch/1
  Constant1/1 -> Product/2  "deltaT"
  Switch1/1 -> X/1
  Constant/1 -> Product/1  "gain"
  Switch/1 -> Y/1, Sum3/2
  R/1 -> Switch1/2, Switch/2
  X/1 -> Switch/3

== system ap_12BAdapted_with_contracts_AutoPilot_SLDV/GlobalScope/DeHavilland Beaver Airframe/Aircraft Dynamics/6DoF (Quaternion)/ResetIntegratorInternal1 ==
  note: ic
  note: Level Reset Integration With Saturation
      | y(n) = y(n-1) + K*Ts*u(n-1)
  U : Inport
  R : Inport  Port=2
  IC : Inport  Port=3
  Constant : Constant  Value=1.0
  Constant1 : Constant  Value=Ts
  Product : Product  RndMeth=Zero
  Product1 : Product  RndMeth=Zero
  Sum3 : Sum
  Switch : Switch  Criteria=u2 ~= 0
  Switch1 : Switch  Criteria=u2 ~= 0
  X : UnitDelay  SampleTime=Ts  HasFrameUpgradeWarning=on
  Y : Outport  VectorParamsAs1DForOutWhenUnconnected=off
  wires:
  Product1/1 -> Sum3/1
  U/1 -> Product1/2
  Sum3/1 -> Switch1/3
  Product/1 -> Product1/1
  IC/1 -> Switch1/1, Switch/1
  Constant1/1 -> Product/2  "deltaT"
  Switch1/1 -> X/1
  Constant/1 -> Product/1  "gain"
  Switch/1 -> Y/1, Sum3/2
  R/1 -> Switch1/2, Switch/2
  X/1 -> Switch/3

== system ap_12BAdapted_with_contracts_AutoPilot_SLDV/GlobalScope/DeHavilland Beaver Airframe/Aircraft Dynamics/6DoF (Quaternion)/ResetIntegratorInternal2 ==
  note: Level Reset Integration With Saturation
      | y(n) = y(n-1) + K*Ts*u(n-1)
  note: ic
  U : Inport
  R : Inport  Port=2
  IC : Inport  Port=3
  Constant : Constant  Value=1.0
  Constant1 : Constant  Value=Ts
  Product : Product  RndMeth=Zero
  Product1 : Product  RndMeth=Zero
  Sum3 : Sum
  Switch : Switch  Criteria=u2 ~= 0
  Switch1 : Switch  Criteria=u2 ~= 0
  X : UnitDelay  SampleTime=Ts  HasFrameUpgradeWarning=on
  Y : Outport  VectorParamsAs1DForOutWhenUnconnected=off
  wires:
  X/1 -> Switch/3
  R/1 -> Switch/2, Switch1/2
  Constant/1 -> Product/1  "gain"
  Switch1/1 -> X/1
  Constant1/1 -> Product/2  "deltaT"
  IC/1 -> Switch/1, Switch1/1
  Product/1 -> Product1/1
  Sum3/1 -> Switch1/3
  U/1 -> Product1/2
  Product1/1 -> Sum3/1
  Switch/1 -> Sum3/2, Y/1

== system ap_12BAdapted_with_contracts_AutoPilot_SLDV/GlobalScope/DeHavilland Beaver Airframe/Aircraft Dynamics/6DoF (Quaternion)/Subsystem ==
  Vb : Inport
  forces : Inport  Port=2
  "mass " : Inport  Port=3
  m_dot : Inport  Port=4  OutDataTypeStr=double
  I : Inport  Port=5  OutDataTypeStr=double
  I_dot : Inport  Port=6  OutDataTypeStr=double
  Constant : Constant  Value=beaver_mass  OutDataTypeStr=Inherit: Inherit via back propagation
  Constant1 : Constant  Value=[inertia; zeros(3,3)]  OutDataTypeStr=Inherit: Inherit via back propagation
  Ground : Ground
  Terminator{,1..4} (5 alike) : Terminator
  "forces " : Outport  VectorParamsAs1DForOutWhenUnconnected=off
  mass : Outport  Port=2  VectorParamsAs1DForOutWhenUnconnected=off
  "inertia, 0" : Outport  Port=3  VectorParamsAs1DForOutWhenUnconnected=off
  Out9 : Outport  Port=4  VectorParamsAs1DForOutWhenUnconnected=off
  wires:
  Constant1/1 -> "inertia, 0"/1
  "mass "/1 -> Terminator3/1
  forces/1 -> "forces "/1
  Vb/1 -> Terminator4/1
  Constant/1 -> mass/1
  I_dot/1 -> Terminator2/1
  I/1 -> Terminator/1
  Ground/1 -> Out9/1
  m_dot/1 -> Terminator1/1

== system ap_12BAdapted_with_contracts_AutoPilot_SLDV/GlobalScope/DeHavilland Beaver Airframe/Aircraft Dynamics/6DoF (Quaternion)/ic1 ==
  Constant : Constant  Value=0
  Constant1 : Constant  Value=xme_0
  Unit Delay : UnitDelay  InitialCondition=1  SampleTime=-1  HasFrameUpgradeWarning=on
  R : Outport  VectorParamsAs1DForOutWhenUnconnected=off
  IC : Outport  Port=2  VectorParamsAs1DForOutWhenUnconnected=off
  wires:
  Constant/1 -> Unit Delay/1
  Unit Delay/1 -> R/1
  Constant1/1 -> IC/1

== system ap_12BAdapted_with_contracts_AutoPilot_SLDV/GlobalScope/DeHavilland Beaver Airframe/Aircraft Dynamics/6DoF (Quaternion)/ic2 ==
  Constant : Constant  Value=0
  Constant1 : Constant  Value=[44.54;2.714;5.836]
  Unit Delay : UnitDelay  InitialCondition=1  SampleTime=-1  HasFrameUpgradeWarning=on
  R : Outport  VectorParamsAs1DForOutWhenUnconnected=off
  IC : Outport  Port=2  VectorParamsAs1DForOutWhenUnconnected=off
  wires:
  Constant1/1 -> IC/1
  Constant/1 -> Unit Delay/1
  Unit Delay/1 -> R/1

== system ap_12BAdapted_with_contracts_AutoPilot_SLDV/GlobalScope/DeHavilland Beaver Airframe/Aircraft Dynamics/6DoF (Quaternion)/ic3 ==
  Constant : Constant  Value=0
  Constant1 : Constant  Value=0
  Unit Delay : UnitDelay  InitialCondition=1  SampleTime=-1  HasFrameUpgradeWarning=on
  R : Outport  VectorParamsAs1DForOutWhenUnconnected=off
  IC : Outport  Port=2  VectorParamsAs1DForOutWhenUnconnected=off
  wires:
  Constant/1 -> Unit Delay/1
  Unit Delay/1 -> R/1
  Constant1/1 -> IC/1

== system ap_12BAdapted_with_contracts_AutoPilot_SLDV/GlobalScope/DeHavilland Beaver Airframe/Aircraft Dynamics/6DoF (Quaternion)/transform to Inertial axes  ==
  x y z : Inport
  transform coefficients : Inport  Port=2
  Product : Product  Multiplication=Matrix(*)  SaturateOnIntegerOverflow=on  InputSameDT=on  OutDataTypeStr=Inherit: Same as first input
  Reshape1 : Reshape  OutputDimensionality=Column vector (2-D)
  Reshape2 : Reshape
  Ve : Outport  VectorParamsAs1DForOutWhenUnconnected=off
  wires:
  Product/1 -> Reshape2/1
  x y z/1 -> Reshape1/1
  transform coefficients/1 -> Product/1
  Reshape1/1 -> Product/2
  Reshape2/1 -> Ve/1

== system ap_12BAdapted_with_contracts_AutoPilot_SLDV/GlobalScope/DeHavilland Beaver Airframe/Aircraft Dynamics/Total Forces and Moments/Actuators ==
  Pilot : Inport
  Bus Selector2 : BusSelector  OutputSignals=uaero
  Demux : Demux
  Initial inputs for aero : Constant  Value=uaero0
  Mux : Mux
  Scope : Scope
  Sum1 : Sum  Inputs=++|  SaturateOnIntegerOverflow=on  InputSameDT=on  OutDataTypeStr=Inherit: Same as first input
  sof : Subsystem
  sof1 : Subsystem
  sof2 : Subsystem
  uaero-out : Outport  VectorParamsAs1DForOutWhenUnconnected=off
  wires:
  Pilot/1 -> Bus Selector2/1
  Initial inputs for aero/1 -> Sum1/1
  Demux/4 -> Mux/4
  Demux/1 -> sof/1(Ac_dem)
  Demux/2 -> sof1/1(Ac_dem)
  Sum1/1 -> Demux/1
  sof/1(Ac_ac) -> Mux/1
  sof1/1(Ac_ac) -> Mux/2
  Bus Selector2/1 -> Sum1/2  "<uaero>"
  Mux/1 -> Scope/1, uaero-out/1
  Demux/3 -> sof2/1(Ac_dem)
  sof2/1(Ac_ac) -> Mux/3

== system ap_12BAdapted_with_contracts_AutoPilot_SLDV/GlobalScope/DeHavilland Beaver Airframe/Aircraft Dynamics/Total Forces and Moments/Aerodynamics ==
  Uaero : Inport
  FltParams : Inport  Port=2
  Actuator Increments : Subsystem
  Body Rate Damping : Subsystem
  Bus Selector1 : BusSelector  OutputSignals=alpha,beta
  Bus Selector2 : BusSelector  OutputSignals=V,pqr_tot
  Datum Coefficients : Subsystem
  Sum1 : Sum  Inputs=|++  SaturateOnIntegerOverflow=on
  Sum4 : Sum  Inputs=|++  SaturateOnIntegerOverflow=on
  Aero Coefficients : Outport  VectorParamsAs1DForOutWhenUnconnected=off
  wires:
  Bus Selector1/2 -> Actuator Increments/2(beta), Datum Coefficients/2(beta)  "<beta>"
  Bus Selector2/1 -> Body Rate Damping/1(V)  "<V>"
  Bus Selector2/2 -> Body Rate Damping/2(p,q,r)  "<pqr_tot>"
  Uaero/1 -> Actuator Increments/3(Actuator Deflections)
  Bus Selector1/1 -> Actuator Increments/1(alpha), Datum Coefficients/1(alpha)  "<alpha>"
  FltParams/1 -> Bus Selector1/1, Bus Selector2/1
  Datum Coefficients/1(Coefficients) -> Sum4/1
  Actuator Increments/1(Coefficients) -> Sum4/2
  Sum4/1 -> Sum1/1
  Body Rate Damping/1(Coefficients) -> Sum1/2
  Sum1/1 -> Aero Coefficients/1

== system ap_12BAdapted_with_contracts_AutoPilot_SLDV/GlobalScope/DeHavilland Beaver Airframe/Aircraft Dynamics/Total Forces and Moments/Engine  ==
  Fltparams : Inport
  Pilot : Inport  Port=2
  rho : Inport  Port=3
  Bus Selector4 : BusSelector  OutputSignals=V,alpha
  eng : Subsystem
  pow : Subsystem
  Engine Coefficients : Outport  VectorParamsAs1DForOutWhenUnconnected=off
  wires:
  Bus Selector4/1 -> pow/3(V)  "<V>"
  rho/1 -> pow/1(rho)
  Bus Selector4/2 -> eng/2(alpha)  "<alpha>"
  eng/1(Cprop) -> Engine Coefficients/1
  Pilot/1 -> pow/2(Pilot)
  pow/1(dpt) -> eng/1(dpt)
  Fltparams/1 -> Bus Selector4/1

== system ap_12BAdapted_with_contracts_AutoPilot_SLDV/GlobalScope/DeHavilland Beaver Airframe/Aircraft Dynamics/Total Forces and Moments/Forces and Moments ==
  Aero Coefficients : Inport
  Fltparams : Inport  Port=2
  Engine Coefficients : Inport  Port=3
  Aero F&M : Subsystem
  Bus Selector4 : BusSelector  OutputSignals=Qdyn
  Scope : Scope
  Sum : Sum  Inputs=++|  SaturateOnIntegerOverflow=on  InputSameDT=on  OutDataTypeStr=Inherit: Same as first input
  neglect center of gravity and center of pressure effects : Constant  Value=[0 0 0]
  XYZ : Outport  VectorParamsAs1DForOutWhenUnconnected=off
  LMN : Outport  Port=2  VectorParamsAs1DForOutWhenUnconnected=off
  wires:
  Sum/1 -> Aero F&M/1(Coefficients)
  Aero Coefficients/1 -> Sum/2
  Engine Coefficients/1 -> Sum/1
  Fltparams/1 -> Bus Selector4/1
  Aero F&M/1(Forces) -> XYZ/1
  neglect center of gravity and center of pressure effects/1 -> Aero F&M/4(CP), Aero F&M/3(CG)
  Bus Selector4/1 -> Scope/1, Aero F&M/2(qbar)  "<Qdyn>"
  Aero F&M/2(Moments) -> LMN/1

== system ap_12BAdapted_with_contracts_AutoPilot_SLDV/GlobalScope/DeHavilland Beaver Airframe/Aircraft Dynamics/Total Forces and Moments/Gravity  ==
  g : Inport
  DCM : Inport  Port=2
  Constant : Constant  Value=0.0
  Gain : Gain  Gain=beaver_mass
  Inertial to Body : Product  Multiplication=Matrix(*)  SaturateOnIntegerOverflow=on  InputSameDT=on  OutDataTypeStr=Inherit: Same as first input
  Mux : Mux  Inputs=3
  Reshape1 : Reshape
  Fgrav : Outport  VectorParamsAs1DForOutWhenUnconnected=off
  wires:
  Inertial to Body/1 -> Reshape1/1
  g/1 -> Gain/1
  DCM/1 -> Inertial to Body/1
  Mux/1 -> Inertial to Body/2
  Reshape1/1 -> Fgrav/1
  Constant/1 -> Mux/2, Mux/1
  Gain/1 -> Mux/3

== system ap_12BAdapted_with_contracts_AutoPilot_SLDV/GlobalScope/DeHavilland Beaver Airframe/Calculate Parameters/ Incidence, Sideslip, & Airspeed/Subsystem ==
  V : Inport
  Demux1 : Demux  Outputs=3
  Terminator : Terminator
  w : Outport  VectorParamsAs1DForOutWhenUnconnected=off
  U : Outport  Port=2  VectorParamsAs1DForOutWhenUnconnected=off
  wires:
  Demux1/3 -> w/1
  Demux1/2 -> Terminator/1
  V/1 -> Demux1/1
  Demux1/1 -> U/1

== system ap_12BAdapted_with_contracts_AutoPilot_SLDV/GlobalScope/DeHavilland Beaver Airframe/Calculate Parameters/ Incidence, Sideslip, & Airspeed/Subsystem1 ==
  V : Inport
  Demux1 : Demux  Outputs=3
  Terminator : Terminator
  Terminator1 : Terminator
  v : Outport  VectorParamsAs1DForOutWhenUnconnected=off
  wires:
  Demux1/1 -> Terminator/1
  Demux1/3 -> Terminator1/1
  V/1 -> Demux1/1
  Demux1/2 -> v/1

== system ap_12BAdapted_with_contracts_AutoPilot_SLDV/GlobalScope/DeHavilland Beaver Airframe/Calculate Parameters/ Incidence, Sideslip, & Airspeed/dot ==
  Vb : Inport
  Demux1 : Demux  Outputs=3
  Product : Product  RndMeth=Zero
  Product1 : Product  RndMeth=Zero
  Product2 : Product  RndMeth=Zero
  Sum : Sum  Inputs=+++
  dot : Outport  VectorParamsAs1DForOutWhenUnconnected=off
  wires:
  Product2/1 -> Sum/3
  Demux1/3 -> Product2/2, Product2/1
  Product/1 -> Sum/1
  Product1/1 -> Sum/2
  Sum/1 -> dot/1
  Vb/1 -> Demux1/1
  Demux1/1 -> Product/2, Product/1
  Demux1/2 -> Product1/1, Product1/2

== system ap_12BAdapted_with_contracts_AutoPilot_SLDV/GlobalScope/DeHavilland Beaver Airframe/Calculate Parameters/Dynamic Pressure/dot ==
  V : Inport
  Demux1 : Demux  Outputs=3
  Product : Product  RndMeth=Zero
  Product1 : Product  RndMeth=Zero
  Product2 : Product  RndMeth=Zero
  Sum : Sum  Inputs=+++
  dot : Outport  VectorParamsAs1DForOutWhenUnconnected=off
  wires:
  Product2/1 -> Sum/3
  Demux1/3 -> Product2/2, Product2/1
  Product/1 -> Sum/1
  Product1/1 -> Sum/2
  Sum/1 -> dot/1
  V/1 -> Demux1/1
  Demux1/1 -> Product/2, Product/1
  Demux1/2 -> Product1/1, Product1/2

== system ap_12BAdapted_with_contracts_AutoPilot_SLDV/GlobalScope/Sensors/Air Data Sensor/ Incidence, Sideslip, & Airspeed/Subsystem ==
  V : Inport
  Demux1 : Demux  Outputs=3
  Terminator : Terminator
  w : Outport  VectorParamsAs1DForOutWhenUnconnected=off
  U : Outport  Port=2  VectorParamsAs1DForOutWhenUnconnected=off
  wires:
  Demux1/3 -> w/1
  Demux1/2 -> Terminator/1
  V/1 -> Demux1/1
  Demux1/1 -> U/1

== system ap_12BAdapted_with_contracts_AutoPilot_SLDV/GlobalScope/Sensors/Air Data Sensor/ Incidence, Sideslip, & Airspeed/Subsystem1 ==
  V : Inport
  Demux1 : Demux  Outputs=3
  Terminator : Terminator
  Terminator1 : Terminator
  v : Outport  VectorParamsAs1DForOutWhenUnconnected=off
  wires:
  Demux1/1 -> Terminator/1
  Demux1/3 -> Terminator1/1
  V/1 -> Demux1/1
  Demux1/2 -> v/1

== system ap_12BAdapted_with_contracts_AutoPilot_SLDV/GlobalScope/Sensors/Air Data Sensor/ Incidence, Sideslip, & Airspeed/dot ==
  Vb : Inport
  Demux1 : Demux  Outputs=3
  Product : Product  RndMeth=Zero
  Product1 : Product  RndMeth=Zero
  Product2 : Product  RndMeth=Zero
  Sum : Sum  Inputs=+++
  dot : Outport  VectorParamsAs1DForOutWhenUnconnected=off
  wires:
  Product2/1 -> Sum/3
  Demux1/3 -> Product2/2, Product2/1
  Product/1 -> Sum/1
  Product1/1 -> Sum/2
  Sum/1 -> dot/1
  Vb/1 -> Demux1/1
  Demux1/1 -> Product/2, Product/1
  Demux1/2 -> Product1/1, Product1/2

== system ap_12BAdapted_with_contracts_AutoPilot_SLDV/GlobalScope/DeHavilland Beaver Airframe/Aircraft Dynamics/6DoF (Quaternion)/3x3 CrossProduct/Subsystem ==
  A : Inport
  B : Inport  Port=2
  Demux : Demux  Outputs=3
  Demux1 : Demux  Outputs=3
  Mux : Mux  Inputs=3
  i x j : Product  SaturateOnIntegerOverflow=on  InputSameDT=on  OutDataTypeStr=Inherit: Same as first input
  j x k : Product  SaturateOnIntegerOverflow=on  InputSameDT=on  OutDataTypeStr=Inherit: Same as first input
  k x i : Product  SaturateOnIntegerOverflow=on  InputSameDT=on  OutDataTypeStr=Inherit: Same as first input
  Out1 : Outport  VectorParamsAs1DForOutWhenUnconnected=off
  wires:
  Demux1/3 -> j x k/2
  Demux/2 -> j x k/1
  Demux/3 -> k x i/1
  Demux1/1 -> k x i/2
  Demux1/2 -> i x j/2
  Demux/1 -> i x j/1
  i x j/1 -> Mux/3
  k x i/1 -> Mux/2
  j x k/1 -> Mux/1
  B/1 -> Demux1/1
  A/1 -> Demux/1
  Mux/1 -> Out1/1

== system ap_12BAdapted_with_contracts_AutoPilot_SLDV/GlobalScope/DeHavilland Beaver Airframe/Aircraft Dynamics/6DoF (Quaternion)/3x3 CrossProduct/Subsystem1 ==
  A : Inport
  B : Inport  Port=2
  Demux : Demux  Outputs=3
  Demux1 : Demux  Outputs=3
  Mux : Mux  Inputs=3
  i x k : Product  SaturateOnIntegerOverflow=on  InputSameDT=on  OutDataTypeStr=Inherit: Same as first input
  j x i : Product  SaturateOnIntegerOverflow=on  InputSameDT=on  OutDataTypeStr=Inherit: Same as first input
  k x j : Product  SaturateOnIntegerOverflow=on  InputSameDT=on  OutDataTypeStr=Inherit: Same as first input
  Out1 : Outport  VectorParamsAs1DForOutWhenUnconnected=off
  wires:
  j x i/1 -> Mux/3
  i x k/1 -> Mux/2
  k x j/1 -> Mux/1
  Mux/1 -> Out1/1
  Demux1/1 -> j x i/2
  Demux/2 -> j x i/1
  Demux1/3 -> i x k/2
  Demux/1 -> i x k/1
  Demux1/2 -> k x j/2
  Demux/3 -> k x j/1
  B/1 -> Demux1/1
  A/1 -> Demux/1
